simulink model "ARC_DTm"  (R2025b)
settings: Solver=FixedStepAuto  StartTime=0.0  StopTime=10080  FixedStep=1  RelTol=1e-3
PreLoadFcn:
  | %For Preload, set the working path
  | modelFolder = fileparts(which(bdroot));
  | addpath(genpath(modelFolder));
StartFcn:
  | tic
StopFcn:
  | fprintf("Sim Time: %.02f min", toc/60)
values from neighbouring files (symbols this model uses):
  batteryScenario = p.batteryScenario    [RUNSIM_ParameterSweep.m]    (also in _RUNSIM_ParameterSweep.m)
  Electricity_SalePriceModifier = 50/100    (= 0.5)    [RUNSIM_ParameterSweep.m]    (also in _RUNSIM_ParameterSweep.m)
  LUT = LUT_load.gamLUT    [RUNSIM_ParameterSweep.m]    (also in _RUNSIM_ParameterSweep.m)
  minimum_UF_system_flow = 5833    [RUNSIM_ParameterSweep.m]    (also in _RUNSIM_ParameterSweep.m)
  PROS1_recoveryrate = 61    [RUNSIM_ParameterSweep.m]    (also in _RUNSIM_ParameterSweep.m)
  PROS2_recoveryrate = 62    [RUNSIM_ParameterSweep.m]    (also in _RUNSIM_ParameterSweep.m)
  ROstabilization_time = p.ROstabilization_time    [RUNSIM_ParameterSweep.m]    (also in _RUNSIM_ParameterSweep.m)
  solarModifier = maximum_solar_generation / 300    [RUNSIM_ParameterSweep.m]    (also in _RUNSIM_ParameterSweep.m)
  TSRO_recoveryrate = 51    [RUNSIM_ParameterSweep.m]    (also in _RUNSIM_ParameterSweep.m)
  UF_RecoveryRate = 96    [RUNSIM_ParameterSweep.m]    (also in _RUNSIM_ParameterSweep.m)
undefined symbols (not defined in the file or in its folder): A_PROS1, A_PROS2, A_TSRO, B_PROS1, B_PROS2, B_TSRO, BW_Max_Time, BW_Max_Vol_gal, CEB_Max_Time, CEB_Max_Vol_gal, CIP_Max_Time, E, FF, h, L, w
libraries: simulink x40
(part 4 of 11)

== system ARC_DTm/TSRO_2 ==
  note: Units needed:
      | u = cm/sec
      | dh = cm
      | Concentrations = g/L
      | Jw_prev = L/m2/min
      |  = Q (Lpm) / Atot(m2)
      | T = oC
      | q = cm/sec =
      | Q (m3/sec) / Atot (m2)
  Inflow : Inport
  Brine Flow (gpm) : Sum  Inputs=-+
  Bus Creator : BusCreator  Inputs=2
  Bus Creator1 : BusCreator  Inputs=3
  Bus Selector : BusSelector  OutputSignals=TSRO Feed Pressure _Bar,Feed Temperature (oC),TSRO_FeedTDS_gL,TSRO_2_FeedFlow_gpm
  Bus Selector1 : BusSelector  OutputSignals=TSRO_A,TSRO_B,TSRO_Area_m2
  Channel Area (m2) : Product  Inputs=4
  Check Valve : Saturate  UpperLimit=Inf  LowerLimit=0
  Check Valve1 : Saturate  UpperLimit=Inf  LowerLimit=0
  Elements per Vessel : Constant  Value=7
  Feed Channel Height (m) : Constant  Value=L
  Fouling Factor : Constant  Value=1-FF
  Gain : Gain  Gain=3.785
  Initial units : Gain  Gain=10^-8
  Jw_Previous : Memory  InitialCondition=.2949
  "L -> gal" : Gain  Gain=1/3.785
  L>m3 : Gain  Gain=1/1000
  MATLAB Function1 : MATLAB Function  TreatAsAtomicUnit=on
  MATLAB Function2 : MATLAB Function  TreatAsAtomicUnit=on
  Membrane Width (m) : Constant  Value=w
  Min : MinMax  Inputs=2
  Minus : Sum  Inputs=+-|
  Number of Vessels : Constant  Value=15
  Pa > Bar : Gain  Gain=100000
  Permeate Flow (gpm) : Product
  Product : Product  Inputs=*/
  Product2 : Product
  Q (L/min) : Gain  Gain=3.785
  Saturation : Saturate  UpperLimit=Inf  LowerLimit=0
  Scope : Scope
      settings: ActiveDisplayYMinimum=-1  ActiveDisplayYMaximum=1  DataLoggingVariableName=ScopeData76
  Scope1 : Scope
      settings: ActiveDisplayYMinimum=-188.84815571077934  ActiveDisplayYMaximum=426.44465787754609  DataLoggingVariableName=ScopeData31
  Scope2 : Scope
      settings: ActiveDisplayYMinimum=-90.1269420343778  ActiveDisplayYMaximum=348.14455140240847  DataLoggingVariableName=ScopeData32
  Spacer Thickness (mm) : Constant  Value=h
  Subsystem : Subsystem
  bar>psi : Gain  Gain=1/.069
  cperm_previous : Memory  InitialCondition=.008
  gpm > L : Gain  Gain=3.785
  initial Units : Gain  Gain=10^-11
  m/min > cm/sec : Gain  Gain=100/60
  m3 > L : Gain  Gain=1000
  m3 > L1 : Gain  Gain=1000
  m>cm : Gain  Gain=100
  m>mm : Gain  Gain=1000
  mm>  cm : Gain  Gain=.1
  mm>m : Gain  Gain=.001
  psi to Bar : Gain  Gain=.069
  s > min : Gain  Gain=60
  s > min1 : Gain  Gain=60
  TSRO_Permeate : Outport
  TSRO_Brine : Outport  Port=2
  tag scope: TSRO_2_deltaPi=global
  wires:
  m/min > cm/sec/1 -> Subsystem/11(u)
  [TSRO_MembraneConstants] -> Bus Selector1/1
  m3 > L1/1 -> s > min1/1
  Bus Selector/1 -> Min/1, Scope/1, bar>psi/1, Subsystem/2(<S2 Feed Pressure (bar)>)  "<TSRO Feed Pressure _Bar>"
  Bus Selector1/3 -> Permeate Flow (gpm)/2  "<TSRO_Area_m2>"
  Membrane Width (m)/1 -> Channel Area (m2)/1, m>mm/1
  [RO_PermeatePressure] -> psi to Bar/1  "Permeate Pressure (psi)"
  Inflow/1 -> Bus Selector/1
  Bus Selector1/1 -> initial Units/1  "<TSRO_A>"
  Bus Selector1/2 -> Initial units/1  "<TSRO_B>"
  Permeate Flow (gpm)/1 -> Check Valve/1  "TSRO_2_PermeateFlow_gpm"
  Bus Selector/2 -> Subsystem/1(<Feed Temperature (oC)>)  "<Feed Temperature (oC)>"
  Bus Selector/3 -> MATLAB Function2/5(cfeed), Subsystem/6(<S2 Feed Salinity (g/L)>)  "<TSRO_FeedTDS_gL>"
  Bus Selector/4 -> Brine Flow (gpm)/2, Q (L/min)/1  "<TSRO_2_FeedFlow_gpm>"
  Product/1 -> m/min > cm/sec/1
  psi to Bar/1 -> Min/2  "Pressure (bar)"
  MATLAB Function2/1(cbrine) -> Bus Creator1/2  "TSRO_2_BrineConductivity_gL"
  initial Units/1 -> m3 > L/1
  Initial units/1 -> m3 > L1/1
  Spacer Thickness (mm)/1 -> MATLAB Function1/2(h), mm>m/1
  m3 > L/1 -> s > min/1
  Min/1 -> Subsystem/3(Pperm)
  mm>m/1 -> Channel Area (m2)/2
  Channel Area (m2)/1 -> Product/2
  Q (L/min)/1 -> MATLAB Function2/4(Qfeed), L>m3/1  "Qtot (L/min)"
  Bus Creator/1 -> Scope2/1, TSRO_Permeate/1  "PRO1_PermeateFlow"
  Number of Vessels/1 -> Channel Area (m2)/3
  s > min/1 -> Pa > Bar/1
  Elements per Vessel/1 -> Channel Area (m2)/4
  s > min1/1 -> Subsystem/5(Salt Perm (L/m2/min))  "Salt Perm (L/m2/min)"
  Fouling Factor/1 -> Product2/2
  m>mm/1 -> MATLAB Function1/1(W)
  L>m3/1 -> Product/1
  Pa > Bar/1 -> Product2/1  "Water Perm (L/m2/min/Bar)"
  MATLAB Function1/1(dh) -> mm>  cm/1
  Feed Channel Height (m)/1 -> m>cm/1
  Jw_Previous/1 -> Subsystem/8(Jw)  "Jw"
  cperm_previous/1 -> Subsystem/7(cperm)  "cperm"
  m>cm/1 -> Subsystem/10(L)
  Product2/1 -> Subsystem/4(Water Perm (L/m2/min/Bar))  "Water Perm (L/m2/min/Bar)"
  Gain/1 -> MATLAB Function2/2(Qperm)  "Predicted Permeate Flow (L/min)"
  mm>  cm/1 -> Subsystem/9(dh)
  Bus Creator1/1 -> Scope1/1, TSRO_Brine/1  "TSRO_Feedwater"
  bar>psi/1 -> Minus/1  "TSRO_2_ConcentratePressure_psi"
  Subsystem/1(Permeate Flux Rate (L/min/m2)) -> Jw_Previous/1, "L -> gal"/1  "Permeate Flux Rate* (L/min.m2)"
  Subsystem/2(Permeate Salinity g/L) -> Bus Creator/2, MATLAB Function2/1(cperm), cperm_previous/1  "TSRO_2_PermeateSalinity_gL"
  "L -> gal"/1 -> Permeate Flow (gpm)/1
  Subsystem/3(deltaPi_bar) -> [TSRO_2_deltaPi]
  Brine Flow (gpm)/1 -> Check Valve1/1  "TSRO_2_BrineFlow_gpm"
  gpm > L/1 -> MATLAB Function2/3(Qbrine)
  [TSRO_Suction_PressureDrop_psi] -> Minus/2
  Minus/1 -> Bus Creator1/3  "TSRO_2_ConcentratePressure_psi"
  Check Valve1/1 -> Bus Creator1/1, gpm > L/1  "TSRO_2_BrineFlow_gpm"
  Check Valve/1 -> Brine Flow (gpm)/1, Bus Creator/1, Gain/1  "TSRO_2_PermeateFlow_gpm"

== system ARC_DTm/TSRO_3 ==
  note: Units needed:
      | u = cm/sec
      | dh = cm
      | Concentrations = g/L
      | Jw_prev = L/m2/min
      |  = Q (Lpm) / Atot(m2)
      | T = oC
      | q = cm/sec =
      | Q (m3/sec) / Atot (m2)
  Inflow : Inport
  Brine Flow (gpm) : Sum  Inputs=-+
  Bus Creator : BusCreator  Inputs=2
  Bus Creator1 : BusCreator  Inputs=3
  Bus Selector : BusSelector  OutputSignals=TSRO Feed Pressure _Bar,Feed Temperature (oC),TSRO_FeedTDS_gL,TSRO_3_FeedFlow_gpm
  Bus Selector1 : BusSelector  OutputSignals=TSRO_A,TSRO_B,TSRO_Area_m2
  Channel Area (m2) : Product  Inputs=4
  Check Valve : Saturate  UpperLimit=Inf  LowerLimit=0
  Check Valve1 : Saturate  UpperLimit=Inf  LowerLimit=0
  Elements per Vessel : Constant  Value=7
  Feed Channel Height (m) : Constant  Value=L
  Fouling Factor : Constant  Value=1-FF
  Gain : Gain  Gain=3.785
  Initial units : Gain  Gain=10^-8
  Jw_Previous : Memory  InitialCondition=.2949
  "L -> gal" : Gain  Gain=1/3.785
  L>m3 : Gain  Gain=1/1000
  MATLAB Function1 : MATLAB Function  TreatAsAtomicUnit=on
  MATLAB Function2 : MATLAB Function  TreatAsAtomicUnit=on
  Membrane Width (m) : Constant  Value=w
  Min : MinMax  Inputs=2
  Minus : Sum  Inputs=+-|
  Number of Vessels : Constant  Value=15
  Pa > Bar : Gain  Gain=100000
  Permeate Flow (gpm) : Product
  Product : Product  Inputs=*/
  Product2 : Product
  Q (L/min) : Gain  Gain=3.785
  Scope : Scope
      settings: ActiveDisplayYMinimum=-1  ActiveDisplayYMaximum=1  DataLoggingVariableName=ScopeData76
  Scope1 : Scope
      settings: ActiveDisplayYMinimum=-188.84815571077934  ActiveDisplayYMaximum=426.44465787754609  DataLoggingVariableName=ScopeData31
  Scope2 : Scope
      settings: ActiveDisplayYMinimum=-90.1269420343778  ActiveDisplayYMaximum=348.14455140240847  DataLoggingVariableName=ScopeData32
  Spacer Thickness (mm) : Constant  Value=h
  Subsystem : Subsystem
  bar>psi : Gain  Gain=1/.069
  cperm_previous : Memory  InitialCondition=.008
  gpm > L : Gain  Gain=3.785
  initial Units : Gain  Gain=10^-11
  m/min > cm/sec : Gain  Gain=100/60
  m3 > L : Gain  Gain=1000
  m3 > L1 : Gain  Gain=1000
  m>cm : Gain  Gain=100
  m>mm : Gain  Gain=1000
  mm>  cm : Gain  Gain=.1
  mm>m : Gain  Gain=.001
  psi to Bar : Gain  Gain=.069
  s > min : Gain  Gain=60
  s > min1 : Gain  Gain=60
  TSRO_Permeate : Outport
  TSRO_Brine : Outport  Port=2
  tag scope: TSRO_3_deltaPi=global
  wires:
  m/min > cm/sec/1 -> Subsystem/11(u)
  [TSRO_MembraneConstants] -> Bus Selector1/1
  m3 > L1/1 -> s > min1/1
  Bus Selector/1 -> Min/1, Scope/1, bar>psi/1, Subsystem/2(<S2 Feed Pressure (bar)>)  "<TSRO Feed Pressure _Bar>"
  Bus Selector1/3 -> Permeate Flow (gpm)/2  "<TSRO_Area_m2>"
  Membrane Width (m)/1 -> Channel Area (m2)/1, m>mm/1
  [RO_PermeatePressure] -> psi to Bar/1  "Permeate Pressure (psi)"
  Inflow/1 -> Bus Selector/1
  Bus Selector1/1 -> initial Units/1  "<TSRO_A>"
  Bus Selector1/2 -> Initial units/1  "<TSRO_B>"
  Permeate Flow (gpm)/1 -> Check Valve1/1  "TSRO_3_PermeateFlow_gpm"
  Bus Selector/2 -> Subsystem/1(<Feed Temperature (oC)>)  "<Feed Temperature (oC)>"
  Bus Selector/3 -> MATLAB Function2/5(cfeed), Subsystem/6(<S2 Feed Salinity (g/L)>)  "<TSRO_FeedTDS_gL>"
  Bus Selector/4 -> Brine Flow (gpm)/2, Q (L/min)/1  "<TSRO_3_FeedFlow_gpm>"
  Product/1 -> m/min > cm/sec/1
  psi to Bar/1 -> Min/2  "Pressure (bar)"
  MATLAB Function2/1(cbrine) -> Bus Creator1/2  "TSRO_3_BrineConductivity_gL"
  initial Units/1 -> m3 > L/1
  Initial units/1 -> m3 > L1/1
  Spacer Thickness (mm)/1 -> MATLAB Function1/2(h), mm>m/1
  m3 > L/1 -> s > min/1
  Min/1 -> Subsystem/3(Pperm)
  mm>m/1 -> Channel Area (m2)/2
  Channel Area (m2)/1 -> Product/2
  Q (L/min)/1 -> MATLAB Function2/4(Qfeed), L>m3/1  "Qtot (L/min)"
  Bus Creator/1 -> Scope2/1, TSRO_Permeate/1  "PRO1_PermeateFlow"
  Number of Vessels/1 -> Channel Area (m2)/3
  s > min/1 -> Pa > Bar/1
  Elements per Vessel/1 -> Channel Area (m2)/4
  s > min1/1 -> Subsystem/5(Salt Perm (L/m2/min))  "Salt Perm (L/m2/min)"
  Fouling Factor/1 -> Product2/2
  m>mm/1 -> MATLAB Function1/1(W)
  L>m3/1 -> Product/1
  Pa > Bar/1 -> Product2/1  "Water Perm (L/m2/min/Bar)"
  MATLAB Function1/1(dh) -> mm>  cm/1
  Feed Channel Height (m)/1 -> m>cm/1
  Jw_Previous/1 -> Subsystem/8(Jw)  "Jw"
  cperm_previous/1 -> Subsystem/7(cperm)  "cperm"
  m>cm/1 -> Subsystem/10(L)
  Product2/1 -> Subsystem/4(Water Perm (L/m2/min/Bar))  "Water Perm (L/m2/min/Bar)"
  Gain/1 -> MATLAB Function2/2(Qperm)  "Predicted Permeate Flow (L/min)"
  mm>  cm/1 -> Subsystem/9(dh)
  Bus Creator1/1 -> Scope1/1, TSRO_Brine/1  "TSRO_Feedwater"
  bar>psi/1 -> Minus/1  "TSRO_3_ConcentratePressure_psi"
  Subsystem/1(Permeate Flux Rate (L/min/m2)) -> Jw_Previous/1, "L -> gal"/1  "Permeate Flux Rate* (L/min.m2)"
  Subsystem/2(Permeate Salinity g/L) -> Bus Creator/2, MATLAB Function2/1(cperm), cperm_previous/1  "TSRO_3_PermeateSalinity_gL"
  "L -> gal"/1 -> Permeate Flow (gpm)/1
  Subsystem/3(deltaPi_bar) -> [TSRO_3_deltaPi]
  Check Valve/1 -> gpm > L/1, Bus Creator1/1  "TSRO_3_BrineFlow_gpm"
  gpm > L/1 -> MATLAB Function2/3(Qbrine)
  [TSRO_Suction_PressureDrop_psi] -> Minus/2
  Minus/1 -> Bus Creator1/3  "TSRO_3_ConcentratePressure_psi"
  Brine Flow (gpm)/1 -> Check Valve/1  "TSRO_3_BrineFlow_gpm"
  Check Valve1/1 -> Brine Flow (gpm)/1, Bus Creator/1, Gain/1  "TSRO_3_PermeateFlow_gpm"

== system ARC_DTm/TSRO_4 ==
  note: Units needed:
      | u = cm/sec
      | dh = cm
      | Concentrations = g/L
      | Jw_prev = L/m2/min
      |  = Q (Lpm) / Atot(m2)
      | T = oC
      | q = cm/sec =
      | Q (m3/sec) / Atot (m2)
  Inflow : Inport
  Brine Flow (gpm) : Sum  Inputs=-+
  Bus Creator : BusCreator  Inputs=2
  Bus Creator1 : BusCreator  Inputs=3
  Bus Selector : BusSelector  OutputSignals=TSRO Feed Pressure _Bar,Feed Temperature (oC),TSRO_FeedTDS_gL,TSRO_4_FeedFlow_gpm
  Bus Selector1 : BusSelector  OutputSignals=TSRO_A,TSRO_B,TSRO_Area_m2
  Channel Area (m2) : Product  Inputs=4
  Check Valve : Saturate  UpperLimit=Inf  LowerLimit=0
  Check Valve1 : Saturate  UpperLimit=Inf  LowerLimit=0
  Elements per Vessel : Constant  Value=7
  Feed Channel Height (m) : Constant  Value=L
  Fouling Factor : Constant  Value=1-FF
  Gain : Gain  Gain=3.785
  Initial units : Gain  Gain=10^-8
  Jw_Previous : Memory  InitialCondition=.2949
  "L -> gal" : Gain  Gain=1/3.785
  L>m3 : Gain  Gain=1/1000
  MATLAB Function1 : MATLAB Function  TreatAsAtomicUnit=on
  MATLAB Function2 : MATLAB Function  TreatAsAtomicUnit=on
  Membrane Width (m) : Constant  Value=w
  Min : MinMax  Inputs=2
  Minus : Sum  Inputs=+-|
  Number of Vessels : Constant  Value=15
  Pa > Bar : Gain  Gain=100000
  Permeate Flow (gpm) : Product
  Product : Product  Inputs=*/
  Product2 : Product
  Q (L/min) : Gain  Gain=3.785
  Scope : Scope
      settings: ActiveDisplayYMinimum=-1  ActiveDisplayYMaximum=1  DataLoggingVariableName=ScopeData76
  Scope1 : Scope
      settings: ActiveDisplayYMinimum=-106.05017960921796  ActiveDisplayYMaximum=153.48557143336205  DataLoggingVariableName=ScopeData31
  Scope2 : Scope
      settings: ActiveDisplayYMinimum=-90.1269420343778  ActiveDisplayYMaximum=348.14455140240847  DataLoggingVariableName=ScopeData32
  Spacer Thickness (mm) : Constant  Value=h
  Subsystem : Subsystem
  bar>psi : Gain  Gain=1/.069
  cperm_previous : Memory  InitialCondition=.008
  gpm > L : Gain  Gain=3.785
  initial Units : Gain  Gain=10^-11
  m/min > cm/sec : Gain  Gain=100/60
  m3 > L : Gain  Gain=1000
  m3 > L1 : Gain  Gain=1000
  m>cm : Gain  Gain=100
  m>mm : Gain  Gain=1000
  mm>  cm : Gain  Gain=.1
  mm>m : Gain  Gain=.001
  psi to Bar : Gain  Gain=.069
  s > min : Gain  Gain=60
  s > min1 : Gain  Gain=60
  TSRO_Permeate : Outport
  TSRO_Brine : Outport  Port=2
  tag scope: TSRO_4_deltaPi=global
  wires:
  m/min > cm/sec/1 -> Subsystem/11(u)
  [TSRO_MembraneConstants] -> Bus Selector1/1
  m3 > L1/1 -> s > min1/1
  Bus Selector/1 -> Min/1, Scope/1, bar>psi/1, Subsystem/2(<S2 Feed Pressure (bar)>)  "<TSRO Feed Pressure _Bar>"
  Bus Selector1/3 -> Permeate Flow (gpm)/2  "<TSRO_Area_m2>"
  Membrane Width (m)/1 -> Channel Area (m2)/1, m>mm/1
  [RO_PermeatePressure] -> psi to Bar/1  "Permeate Pressure (psi)"
  Inflow/1 -> Bus Selector/1
  Bus Selector1/1 -> initial Units/1  "<TSRO_A>"
  Bus Selector1/2 -> Initial units/1  "<TSRO_B>"
  Permeate Flow (gpm)/1 -> Check Valve1/1  "TSRO_4_PermeateFlow_gpm"
  Bus Selector/2 -> Subsystem/1(<Feed Temperature (oC)>)  "<Feed Temperature (oC)>"
  Bus Selector/3 -> MATLAB Function2/5(cfeed), Subsystem/6(<S2 Feed Salinity (g/L)>)  "<TSRO_FeedTDS_gL>"
  Bus Selector/4 -> Brine Flow (gpm)/2, Q (L/min)/1  "<TSRO_4_FeedFlow_gpm>"
  Product/1 -> m/min > cm/sec/1
  psi to Bar/1 -> Min/2  "Pressure (bar)"
  MATLAB Function2/1(cbrine) -> Bus Creator1/2  "TSRO_4_BrineConductivity_gL"
  initial Units/1 -> m3 > L/1
  Initial units/1 -> m3 > L1/1
  Spacer Thickness (mm)/1 -> MATLAB Function1/2(h), mm>m/1
  m3 > L/1 -> s > min/1
  Min/1 -> Subsystem/3(Pperm)
  mm>m/1 -> Channel Area (m2)/2
  Channel Area (m2)/1 -> Product/2
  Q (L/min)/1 -> MATLAB Function2/4(Qfeed), L>m3/1  "Qtot (L/min)"
  Bus Creator/1 -> Scope2/1, TSRO_Permeate/1  "PRO1_PermeateFlow"
  Number of Vessels/1 -> Channel Area (m2)/3
  s > min/1 -> Pa > Bar/1
  Elements per Vessel/1 -> Channel Area (m2)/4
  s > min1/1 -> Subsystem/5(Salt Perm (L/m2/min))  "Salt Perm (L/m2/min)"
  Fouling Factor/1 -> Product2/2
  m>mm/1 -> MATLAB Function1/1(W)
  L>m3/1 -> Product/1
  Pa > Bar/1 -> Product2/1  "Water Perm (L/m2/min/Bar)"
  MATLAB Function1/1(dh) -> mm>  cm/1
  Feed Channel Height (m)/1 -> m>cm/1
  Jw_Previous/1 -> Subsystem/8(Jw)  "Jw"
  cperm_previous/1 -> Subsystem/7(cperm)  "cperm"
  m>cm/1 -> Subsystem/10(L)
  Product2/1 -> Subsystem/4(Water Perm (L/m2/min/Bar))  "Water Perm (L/m2/min/Bar)"
  Gain/1 -> MATLAB Function2/2(Qperm)  "Predicted Permeate Flow (L/min)"
  mm>  cm/1 -> Subsystem/9(dh)
  Bus Creator1/1 -> Scope1/1, TSRO_Brine/1  "TSRO_Feedwater"
  bar>psi/1 -> Minus/1  "TSRO_4_ConcentratePressure_psi"
  Subsystem/1(Permeate Flux Rate (L/min/m2)) -> Jw_Previous/1, "L -> gal"/1  "Permeate Flux Rate* (L/min.m2)"
  Subsystem/2(Permeate Salinity g/L) -> Bus Creator/2, MATLAB Function2/1(cperm), cperm_previous/1  "TSRO_4_PermeateSalinity_gL"
  "L -> gal"/1 -> Permeate Flow (gpm)/1
  Subsystem/3(deltaPi_bar) -> [TSRO_4_deltaPi]
  Check Valve/1 -> Bus Creator1/1, gpm > L/1  "TSRO_4_BrineFlow_gpm"
  gpm > L/1 -> MATLAB Function2/3(Qbrine)
  [TSRO_Suction_PressureDrop_psi] -> Minus/2
  Minus/1 -> Bus Creator1/3  "TSRO_4_ConcentratePressure_psi"
  Brine Flow (gpm)/1 -> Check Valve/1  "TSRO_4_BrineFlow_gpm"
  Check Valve1/1 -> Brine Flow (gpm)/1, Bus Creator/1, Gain/1  "TSRO_4_PermeateFlow_gpm"

== system ARC_DTm/TSRO_Pump_1 ==
  note: Determine Needed Added Pressure
  note: gpm / (gpm/psi*ft2) / ft2
  S2 Feed Flow Rate (gpm) : Inport
  Bar > psi : Gain  Gain=1/.069
  Bus Creator : BusCreator  Inputs=4
  Bus Selector : BusSelector  OutputSignals=TSRO_A,TSRO_Area_m2
  Bus Selector1 : BusSelector  OutputSignals=TSRO_1_FeedFlow_gpm,TSRO_FeedTDS_gL,TSRO_SuctionPressure_psi
  Constant : Constant  Value=0
  Display : Display
  Display2 : Display
  Gain3 : Gain  Gain=10.76
  MATLAB Function1 : MATLAB Function  TreatAsAtomicUnit=on
  Max : MinMax  Function=max  Inputs=2
  Memory : Memory
  Pa > psi : Gain  Gain=6895
  Product : Product  Inputs=**/
  Product1 : Product
  Scope : Scope  NumInputPorts=3
      settings: ActiveDisplayYMinimum=410.42447825863661  ActiveDisplayYMaximum=523.485280193485  DataLoggingVariableName=ScopeData21
  Scope1 : Scope  NumInputPorts=4
      settings: ActiveDisplayYMinimum=-70.174712486796437  ActiveDisplayYMaximum=115.33681909060641  DataLoggingVariableName=ScopeData24
  Scope2 : Scope
      settings: ActiveDisplayYMinimum=-1  ActiveDisplayYMaximum=1  DataLoggingVariableName=ScopeData18
  Scope3 : Scope
      settings: ActiveDisplayYMinimum=2.9110767702794598  ActiveDisplayYMaximum=3.7356434036475763  DataLoggingVariableName=ScopeData33
  Sum : Sum  Inputs=|-+
  Sum1 : Sum  Inputs=|++
  Sum2 : Sum  Inputs=|++
  m2 > ft2 : Gain  Gain=1/10.76
  m3 > gal : Gain  Gain=264.2
  m3/m2/s/Pa : Gain  Gain=10^-11
  psi to Bar : Gain  Gain=.069
  psi>ft : Gain  Gain=2.31
  s > min : Gain  Gain=60
  TSRO_1_Feedwater : Outport
  tag scope: TSRO_1_Power_kW=global
  wires:
  S2 Feed Flow Rate (gpm)/1 -> Bus Selector1/1  "InflowRate (gpm)"
  Sum1/1 -> Sum2/1  "Net Opposing Pressure (psi)"
  [TSRO_MembraneConstants] -> Bus Selector/1
  Pa > psi/1 -> m2 > ft2/1  "Water Perm (gpm/m2/bar)"
  Sum2/1 -> psi to Bar/1, Sum/2  "TSRO_1_FeedPressure_psi"
  m3 > gal/1 -> s > min/1
  [RO_PermeatePressure] -> Sum1/2
  [T] -> Bus Creator/2  "Feed Temperature (oC)"
  Memory/1 -> Scope1/3, Sum1/1
  Product/1 -> Sum2/2, Scope1/1  "TSRO_1_RequiredNDP_psi"
  psi to Bar/1 -> Bus Creator/4  "TSRO Feed Pressure _Bar"
  Gain3/1 -> Display/1, Product1/2  "TSRO_Area_ft2"
  m2 > ft2/1 -> Product1/1  "TSRO_WaterPermeability_gpm_psi_ft2"
  m3/m2/s/Pa/1 -> m3 > gal/1
  Bus Selector/1 -> m3/m2/s/Pa/1  "<TSRO_A>"
  Product1/1 -> Product/3
  [TSRO_1_deltaPi] -> Scope2/1, Bar > psi/1
  [TSRO_RR] -> Product/2
  s > min/1 -> Pa > psi/1
  Bar > psi/1 -> Memory/1
  Bus Creator/1 -> TSRO_1_Feedwater/1
  psi>ft/1 -> Scope/2, MATLAB Function1/2(h_des)
  Bus Selector1/2 -> Scope3/1, Bus Creator/1  "<TSRO_FeedTDS_gL>"
  Bus Selector1/3 -> Scope1/2, Sum/1  "<TSRO_SuctionPressure_psi>"
  Bus Selector/2 -> Gain3/1  "<TSRO_Area_m2>"
  Bus Selector1/1 -> MATLAB Function1/1(Q_des), Scope/1, Bus Creator/3, Product/1  "<TSRO_1_FeedFlow_gpm>"
  Sum/1 -> Scope1/4, psi>ft/1  "Required added pressure (psi)"
  Max/1 -> [TSRO_1_Power_kW], Display2/1
  Constant/1 -> Max/1
  MATLAB Function1/1(power) -> Max/2, Scope/3  "TSRO_1_Power_kW"

== system ARC_DTm/TSRO_Pump_2 ==
  note: Determine Needed Added Pressure
  note: gpm / (gpm/psi*ft2) / ft2
  S2 Feed Flow Rate (gpm) : Inport
  Bar > psi : Gain  Gain=1/.069
  Bus Creator : BusCreator  Inputs=4
  Bus Selector : BusSelector  OutputSignals=TSRO_A,TSRO_Area_m2
  Bus Selector1 : BusSelector  OutputSignals=TSRO_2_FeedFlow_gpm,TSRO_FeedTDS_gL,TSRO_SuctionPressure_psi
  Constant : Constant  Value=0
  Display : Display
  Display2 : Display
  Gain : Gain  Gain=.01
  Gain3 : Gain  Gain=10.76
  MATLAB Function1 : MATLAB Function  TreatAsAtomicUnit=on
  Max : MinMax  Function=max  Inputs=2
  Memory : Memory
  Pa > psi : Gain  Gain=6895
  Product : Product  Inputs=**/
  Product1 : Product
  Sum : Sum  Inputs=|-+
  Sum1 : Sum  Inputs=|++
  Sum2 : Sum  Inputs=|++
  TSRO_2_recoveryrate_per : Constant  Value=51
  m2 > ft2 : Gain  Gain=1/10.76
  m3 > gal : Gain  Gain=264.2
  m3/m2/s/Pa : Gain  Gain=10^-11
  psi to Bar : Gain  Gain=.069
  psi>ft : Gain  Gain=2.31
  s > min : Gain  Gain=60
  TSRO_2_Feedwater : Outport
  tag scope: TSRO_2_Power_kW=global
  wires:
  S2 Feed Flow Rate (gpm)/1 -> Bus Selector1/1  "InflowRate (gpm)"
  Sum1/1 -> Sum2/1  "Net Opposing Pressure (psi)"
  [TSRO_MembraneConstants] -> Bus Selector/1
  Pa > psi/1 -> m2 > ft2/1  "Water Perm (gpm/m2/bar)"
  Sum2/1 -> psi to Bar/1, Sum/2  "TSRO_2_FeedPressure_psi"
  m3 > gal/1 -> s > min/1
  [RO_PermeatePressure] -> Sum1/2
  [T] -> Bus Creator/2  "Feed Temperature (oC)"
  Memory/1 -> Sum1/1
  Product/1 -> Sum2/2  "TSRO_2_RequiredNDP_psi"
  TSRO_2_recoveryrate_per/1 -> Gain/1
  psi to Bar/1 -> Bus Creator/4  "TSRO Feed Pressure _Bar"
  Gain3/1 -> Display/1, Product1/2  "TSRO_Area_ft2"
  m2 > ft2/1 -> Product1/1  "TSRO_WaterPermeability_gpm_psi_ft2"
  m3/m2/s/Pa/1 -> m3 > gal/1
  Bus Selector/1 -> m3/m2/s/Pa/1  "<TSRO_A>"
  Product1/1 -> Product/3
  [TSRO_2_deltaPi] -> Bar > psi/1
  Gain/1 -> Product/2
  s > min/1 -> Pa > psi/1
  Bar > psi/1 -> Memory/1
  Bus Creator/1 -> TSRO_2_Feedwater/1
  psi>ft/1 -> MATLAB Function1/2(h_des)
  Bus Selector1/2 -> Bus Creator/1  "<TSRO_FeedTDS_gL>"
  Bus Selector1/3 -> Sum/1  "<TSRO_SuctionPressure_psi>"
  Bus Selector/2 -> Gain3/1  "<TSRO_Area_m2>"
  Bus Selector1/1 -> MATLAB Function1/1(Q_des), Bus Creator/3, Product/1  "<TSRO_2_FeedFlow_gpm>"
  Sum/1 -> psi>ft/1
  Max/1 -> Display2/1, [TSRO_2_Power_kW]
  Constant/1 -> Max/1
  MATLAB Function1/1(power) -> Max/2

== system ARC_DTm/TSRO_Pump_3 ==
  note: Determine Needed Added Pressure
  note: gpm / (gpm/psi*ft2) / ft2
  S2 Feed Flow Rate (gpm) : Inport
  Bar > psi : Gain  Gain=1/.069
  Bus Creator : BusCreator  Inputs=4
  Bus Selector : BusSelector  OutputSignals=TSRO_A,TSRO_Area_m2
  Bus Selector1 : BusSelector  OutputSignals=TSRO_3_FeedFlow_gpm,TSRO_FeedTDS_gL,TSRO_SuctionPressure_psi
  Constant : Constant  Value=0
  Display : Display
  Display2 : Display
  Gain : Gain  Gain=.01
  Gain3 : Gain  Gain=10.76
  MATLAB Function1 : MATLAB Function  TreatAsAtomicUnit=on
  Max : MinMax  Function=max  Inputs=2
  Memory : Memory
  Pa > psi : Gain  Gain=6895
  Product : Product  Inputs=**/
  Product1 : Product
  Sum : Sum  Inputs=|-+
  Sum1 : Sum  Inputs=|++
  Sum2 : Sum  Inputs=|++
  TSRO_3_recoveryrate_per : Constant  Value=51
  m2 > ft2 : Gain  Gain=1/10.76
  m3 > gal : Gain  Gain=264.2
  m3/m2/s/Pa : Gain  Gain=10^-11
  psi to Bar : Gain  Gain=.069
  psi>ft : Gain  Gain=2.31
  s > min : Gain  Gain=60
  TSRO_3_Feedwater : Outport
  tag scope: TSRO_3_Power_kW=global
  wires:
  S2 Feed Flow Rate (gpm)/1 -> Bus Selector1/1  "InflowRate (gpm)"
  Sum1/1 -> Sum2/1  "Net Opposing Pressure (psi)"
  [TSRO_MembraneConstants] -> Bus Selector/1
  Pa > psi/1 -> m2 > ft2/1  "Water Perm (gpm/m2/bar)"
  Sum2/1 -> psi to Bar/1, Sum/2  "TSRO_3_FeedPressure_psi"
  m3 > gal/1 -> s > min/1
  [RO_PermeatePressure] -> Sum1/2
  [T] -> Bus Creator/2  "Feed Temperature (oC)"
  Memory/1 -> Sum1/1
  Product/1 -> Sum2/2  "TSRO_3_RequiredNDP_psi"
  TSRO_3_recoveryrate_per/1 -> Gain/1
  psi to Bar/1 -> Bus Creator/4  "TSRO Feed Pressure _Bar"
  Gain3/1 -> Display/1, Product1/2  "TSRO_Area_ft2"
  m2 > ft2/1 -> Product1/1  "TSRO_WaterPermeability_gpm_psi_ft2"
  m3/m2/s/Pa/1 -> m3 > gal/1
  Bus Selector/1 -> m3/m2/s/Pa/1  "<TSRO_A>"
  Product1/1 -> Product/3
  [TSRO_3_deltaPi] -> Bar > psi/1
  Gain/1 -> Product/2
  s > min/1 -> Pa > psi/1
  Bar > psi/1 -> Memory/1
  Bus Creator/1 -> TSRO_3_Feedwater/1
  psi>ft/1 -> MATLAB Function1/2(h_des)
  Bus Selector1/2 -> Bus Creator/1  "<TSRO_FeedTDS_gL>"
  Bus Selector1/3 -> Sum/1  "<TSRO_SuctionPressure_psi>"
  Bus Selector/2 -> Gain3/1  "<TSRO_Area_m2>"
  Bus Selector1/1 -> MATLAB Function1/1(Q_des), Bus Creator/3, Product/1  "<TSRO_3_FeedFlow_gpm>"
  Sum/1 -> psi>ft/1
  Max/1 -> Display2/1, [TSRO_3_Power_kW]
  Constant/1 -> Max/1
  MATLAB Function1/1(power) -> Max/2

== system ARC_DTm/TSRO_Pump_4 ==
  note: Determine Needed Added Pressure
  note: gpm / (gpm/psi*ft2) / ft2
  S2 Feed Flow Rate (gpm) : Inport
  Bar > psi : Gain  Gain=1/.069
  Bus Creator : BusCreator  Inputs=4
  Bus Selector : BusSelector  OutputSignals=TSRO_A,TSRO_Area_m2
  Bus Selector1 : BusSelector  OutputSignals=TSRO_4_FeedFlow_gpm,TSRO_FeedTDS_gL,TSRO_SuctionPressure_psi
  Constant : Constant  Value=0
  Display : Display
  Display2 : Display
  Gain : Gain  Gain=.01
  Gain3 : Gain  Gain=10.76
  MATLAB Function1 : MATLAB Function  TreatAsAtomicUnit=on
  Max : MinMax  Function=max  Inputs=2
  Memory : Memory
  Pa > psi : Gain  Gain=6895
  Product : Product  Inputs=**/
  Product1 : Product
  Sum : Sum  Inputs=|-+
  Sum1 : Sum  Inputs=|++
  Sum2 : Sum  Inputs=|++
  TSRO_4_recoveryrate_per : Constant  Value=51
  m2 > ft2 : Gain  Gain=1/10.76
  m3 > gal : Gain  Gain=264.2
  m3/m2/s/Pa : Gain  Gain=10^-11
  psi to Bar : Gain  Gain=.069
  psi>ft : Gain  Gain=2.31
  s > min : Gain  Gain=60
  TSRO_4_Feedwater : Outport
  tag scope: TSRO_4_Power_kW=global
  wires:
  S2 Feed Flow Rate (gpm)/1 -> Bus Selector1/1  "InflowRate (gpm)"
  Sum1/1 -> Sum2/1  "Net Opposing Pressure (psi)"
  [TSRO_MembraneConstants] -> Bus Selector/1
  Pa > psi/1 -> m2 > ft2/1  "Water Perm (gpm/m2/bar)"
  Sum2/1 -> psi to Bar/1, Sum/2  "TSRO_4_FeedPressure_psi"
  m3 > gal/1 -> s > min/1
  [RO_PermeatePressure] -> Sum1/2
  [T] -> Bus Creator/2  "Feed Temperature (oC)"
  Memory/1 -> Sum1/1
  Product/1 -> Sum2/2  "TSRO_4_RequiredNDP_psi"
  TSRO_4_recoveryrate_per/1 -> Gain/1
  psi to Bar/1 -> Bus Creator/4  "TSRO Feed Pressure _Bar"
  Gain3/1 -> Display/1, Product1/2  "TSRO_Area_ft2"
  m2 > ft2/1 -> Product1/1  "TSRO_WaterPermeability_gpm_psi_ft2"
  m3/m2/s/Pa/1 -> m3 > gal/1
  Bus Selector/1 -> m3/m2/s/Pa/1  "<TSRO_A>"
  Product1/1 -> Product/3
  [TSRO_4_deltaPi] -> Bar > psi/1
  Gain/1 -> Product/2
  s > min/1 -> Pa > psi/1
  Bar > psi/1 -> Memory/1
  Bus Creator/1 -> TSRO_4_Feedwater/1
  psi>ft/1 -> MATLAB Function1/2(h_des)
  Bus Selector1/2 -> Bus Creator/1  "<TSRO_FeedTDS_gL>"
  Bus Selector1/3 -> Sum/1  "<TSRO_SuctionPressure_psi>"
  Bus Selector/2 -> Gain3/1  "<TSRO_Area_m2>"
  Bus Selector1/1 -> MATLAB Function1/1(Q_des), Bus Creator/3, Product/1  "<TSRO_4_FeedFlow_gpm>"
  Sum/1 -> psi>ft/1
  Max/1 -> Display2/1, [TSRO_4_Power_kW]
  Constant/1 -> Max/1
  MATLAB Function1/1(power) -> Max/2

== system ARC_DTm/UF Maintenance Coordinator ==
  Bus Creator{,1..9} (10 alike) : BusCreator  Inputs=2
  Demux : Demux  Outputs=10
  Demux1 : Demux  Outputs=10
  Maint Queue Vector2 : Mux  Inputs=10
  Memory : Memory
  Memory1 : Memory
  Memory2 : Memory
  Sample_Stateflows : Stateflow chart  Commented=on  TreatAsAtomicUnit=on
  Scope1 : Scope  NumInputPorts=3
      settings: ActiveDisplayYMinimum=-1.25  ActiveDisplayYMaximum=1.25
  Scope2 : Scope
      settings: ActiveDisplayYMinimum=-1  ActiveDisplayYMaximum=1  DataLoggingVariableName=ScopeData14
  Scope3 : Scope
      settings: ActiveDisplayYMinimum=-1  ActiveDisplayYMaximum=1  DataLoggingVariableName=ScopeData15
  Scope5 : Scope
      settings: ActiveDisplayYMinimum=-1.2345292012789748  ActiveDisplayYMaximum=1.3904707987210259  DataLoggingVariableName=ScopeData17
  Scope6 : Scope  NumInputPorts=2
      settings: ActiveDisplayYMinimum=-0.12499999999999997  ActiveDisplayYMaximum=1.125  DataLoggingVariableName=ScopeData18
  UF_FIFO_Coordinator : MATLAB Function  Priority=100  TreatAsAtomicUnit=on  SystemSampleTime=1
  UF_State_Tracker : MATLAB Function  TreatAsAtomicUnit=on  SystemSampleTime=1
  arhive : Subsystem
  tag scope: UF10_State=global, UF1_State=global, UF2_State=global, UF3_State=global, UF4_State=global, UF5_State=global, UF6_State=global, UF7_State=global, UF8_State=global, UF9_State=global, UF_Flow_Assignment=global, UF_Operations_States_vector=global
  wires:
  UF_State_Tracker/3(operations_states) -> Scope5/1, [UF_Operations_States_vector], UF_FIFO_Coordinator/3(operating_states)
  UF_State_Tracker/1(in_startup_queue) -> Scope3/1, UF_FIFO_Coordinator/1(startup_req)
  UF_State_Tracker/2(in_maint_queue) -> Scope2/1, UF_FIFO_Coordinator/2(maint_req)
  UF_State_Tracker/4(maintenance_completion_indicators) -> Scope6/1, Scope1/3, [UF_Maintenance_Completion_Signals]  "Maintenance Completion"
  UF_FIFO_Coordinator/1(startup_cmd) -> Memory/1
  UF_FIFO_Coordinator/2(maint_cmd) -> Memory1/1
  Memory/1 -> UF_State_Tracker/1(startup_cmd)
  Memory1/1 -> UF_State_Tracker/2(maint_cmd)
  UF_FIFO_Coordinator/3(shutdown_cmd) -> Memory2/1
  Memory2/1 -> UF_State_Tracker/3(shutdown_cmd)
  [UF2_Maintenance_Request] -> Maint Queue Vector2/2
  [UF3_Maintenance_Request] -> Maint Queue Vector2/3
  [UF7_Maintenance_Request] -> Maint Queue Vector2/7
  [UF8_Maintenance_Request] -> Maint Queue Vector2/8
  [UF5_Maintenance_Request] -> Maint Queue Vector2/5
  [UF6_Maintenance_Request] -> Maint Queue Vector2/6
  [UF10_Maintenance_Request] -> Maint Queue Vector2/10
  [UF9_Maintenance_Request] -> Maint Queue Vector2/9
  [UF4_Maintenance_Request] -> Maint Queue Vector2/4
  [UF1_Maintenance_Request] -> Maint Queue Vector2/1
  [UF_Maintenance_Completion_Signals] -> Demux/1
  Maint Queue Vector2/1 -> Scope6/2, UF_State_Tracker/4(maint_req)
  Demux/1 -> Bus Creator/1  "UF1_MaintenanceCompletion_signal"
  Bus Creator/1 -> [UF1_State]
  Demux/2 -> Bus Creator1/1  "UF2_MaintenanceCompletion_signal"
  Demux/3 -> Bus Creator2/1  "UF3_MaintenanceCompletion_signal"
  Demux/4 -> Bus Creator3/1  "UF4_MaintenanceCompletion_signal"
  Demux/5 -> Bus Creator4/1  "UF5_MaintenanceCompletion_signal"
  Bus Creator1/1 -> [UF2_State]
  Demux/6 -> Bus Creator5/1  "UF6_MaintenanceCompletion_signal"
  Bus Creator3/1 -> [UF4_State]
  Bus Creator2/1 -> [UF3_State]
  Bus Creator5/1 -> [UF6_State]
  Bus Creator4/1 -> [UF5_State]
  Bus Creator7/1 -> [UF8_State]
  Bus Creator6/1 -> [UF7_State]
  Bus Creator9/1 -> [UF10_State]
  Bus Creator8/1 -> [UF9_State]
  Demux/7 -> Bus Creator6/1  "UF7_MaintenanceCompletion_signal"
  Demux/8 -> Bus Creator7/1  "UF8_MaintenanceCompletion_signal"
  Demux/9 -> Bus Creator8/1  "UF9_MaintenanceCompletion_signal"
  Demux/10 -> Bus Creator9/1  "UF10_MaintenanceCompletion_signal"
  Demux1/2 -> Bus Creator1/2  "UF2_OperationsState_signal"
  Demux1/7 -> Bus Creator6/2  "UF7_OperationsState_signal"
  Demux1/10 -> Bus Creator9/2  "UF10_OperationsState_signal"
  Demux1/1 -> Bus Creator/2  "UF1_OperationsState_signal"
  Demux1/8 -> Bus Creator7/2  "UF8_OperationsState_signal"
  Demux1/4 -> Bus Creator3/2  "UF4_OperationsState_signal"
  Demux1/9 -> Bus Creator8/2  "UF9_OperationsState_signal"
  Demux1/3 -> Bus Creator2/2  "UF3_OperationsState_signal"
  [UF_Operations_States_vector] -> Scope1/1, Demux1/1  "OperationsStates"
  Demux1/5 -> Bus Creator4/2  "UF5_OperationsState_signal"
  Demux1/6 -> Bus Creator5/2  "UF6_OperationsState_signal"
  UF_FIFO_Coordinator/4(assigned_flows) -> Scope1/2, [UF_Flow_Assignment]  "Flows"
  [UFMembrane_FlowVector] -> UF_FIFO_Coordinator/4(flows)

== system ARC_DTm/UF Pumping ==
  Autostrainer_HeadLoss_psi : Constant  Value=5
  Bus Creator : BusCreator  Inputs=3
  Bus Selector : BusSelector  OutputSignals=MaxFlow_gpm,MinFlow_gpm
  Bus Selector1 : BusSelector  OutputSignals=Plant Feed Setpoint,Plant Feed Actual
  Display : Display
  Display1 : Display
  MATLAB Function : MATLAB Function  TreatAsAtomicUnit=on
  Memory : Memory
  Memory1 : Memory
  Saturation : Saturate  UpperLimit=11000  LowerLimit=minimum_UF_system_flow
  Saturation1 : Saturate  UpperLimit=11000  LowerLimit=minimum_UF_system_flow
  Scope : Scope  NumInputPorts=4
      settings: ActiveDisplayYMinimum=-11.154361957059978  ActiveDisplayYMaximum=100.38925761353981  DataLoggingVariableName=ScopeData23
  Sum : Sum  Inputs=+-+|
  Sum1 : Sum  Inputs=|-+
  UF_SuctionPressure_psi : Constant  Value=-12
  psi > ft : Gain  Gain=2.31
  UF_Pump_Discharge : Outport
  tag scope: UFPump_FlowperUnit=global, UF_PumpPower_Vector=global
  wires:
  Sum/1 -> Memory1/1  "UF Feed Pressure_psi"
  UF_SuctionPressure_psi/1 -> Sum/2  "S1 Suction Pressure (psi)"
  MATLAB Function/2(powers) -> [UF_PumpPower_Vector], Scope/2  "Predicted Power Consumption (kW)"
  Bus Creator/1 -> UF_Pump_Discharge/1
  [UFPump_FeedPressure_psi] -> Sum/3
  [UF_FeedFlow] -> Scope/4, Bus Selector1/1
  [UFPump_Bounds] -> Bus Selector/1
  Bus Selector/1 -> MATLAB Function/1(max_flow_per_unit)  "<MaxFlow_gpm>"
  MATLAB Function/1(speeds) -> Display/1, Scope/1
  Autostrainer_HeadLoss_psi/1 -> Sum1/1, Sum/1  "Autostrainer Headloss_psi"
  Sum1/1 -> Bus Creator/3  "UF_FeedPressure_psi"
  MATLAB Function/4(flows) -> Scope/3, Memory/1, [UFPump_FlowperUnit], Display1/1  "UF Flow Vector"
  psi > ft/1 -> MATLAB Function/6(h_des)
  Bus Selector1/1 -> Saturation/1  "<Plant Feed Setpoint>"
  Bus Selector1/2 -> Saturation1/1  "<Plant Feed Actual>"
  Memory/1 -> MATLAB Function/5(prev_flows)
  Bus Selector/2 -> MATLAB Function/2(min_flow_per_unit)  "<MinFlow_gpm>"
  Saturation/1 -> Bus Creator/1, MATLAB Function/3(flow_setpoint)  "UFFeedFlow_Setpoint_gpm"
  Saturation1/1 -> Bus Creator/2, MATLAB Function/4(flow_actual)  "UFFeedFlow_Actual_gpm"
  Memory1/1 -> Sum1/2, psi > ft/1

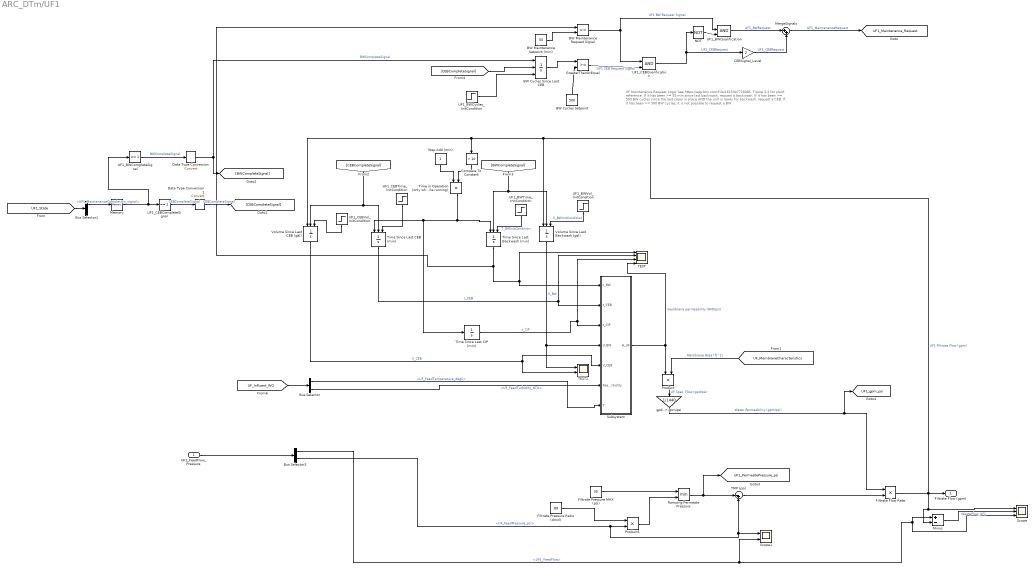
== system ARC_DTm/UF1 ==
  note: UF Maintenance Request Logic
      | See https://app.box.com/file/1615307718366, Figure 3-2 for plant reference.
      |
      | If it has been >= 55 min since last backwash, request a backwash.
      | If it has been >= 500 BW cycles since the last clean in place AND the unit is ready for backwash, request a CEB.
      | If it has been >= 500 BW cycles, it is not possible to request a BW
  UF1_FeedFlow_Pressure : Inport
  BW Cycles Setpoint : Constant  Value=500
  BW Cycles Since Last CEB : Integrator  ExternalReset=rising  InitialConditionSource=external  InitialCondition=5
  BW Maintenance Request Signal : RelationalOperator  OutDataTypeStr=boolean  RndMeth=Simplest  InputSameDT=off
  BW Maintenance Setpoint (min) : Constant  Value=55
  Bus Selector : BusSelector  OutputSignals=UF_FeedTemperature_degC,UF_FeedTurbidity_NTU
  Bus Selector1 : BusSelector  OutputSignals=UF1_MaintenanceCompletion_signal,UF1_OperationsState_signal
  Bus Selector3 : BusSelector  OutputSignals=UF1_FeedFlow,UF_FeedPressure_psi
  CEBSignal_Level : Gain  Gain=2  OutDataTypeStr=double
  Compare To Constant : simulink/Logic and Bit Operations/Compare To Constant  relop=>  const=10  OutDataTypeStr=boolean
  Data Type Conversion : DataTypeConversion  SaturateOnIntegerOverflow=off  RndMeth=Floor
  Data Type Conversion1 : DataTypeConversion  SaturateOnIntegerOverflow=off  RndMeth=Floor
  Filtrate Flow Rate : Product
  Filtrate Pressure MAX (psi) : Constant  Value=39
  Filtrate Pressure Ratio (dmnl) : Constant  Value=.89
  GreaterThanOrEqual : RelationalOperator  OutDataTypeStr=boolean  RndMeth=Simplest  InputSameDT=off
  Memory : Memory
  MergeSignals : Sum  Inputs=|++
  Minus : Sum  Inputs=+-
  NOT : Logic  Operator=NOT  IconShape=distinctive  AllPortsSameDT=off  OutDataTypeStr=boolean
  Product : Product
  Product1 : Product
  Ramping Permeate Pressure : MinMax  Inputs=2
  Scope : Scope  NumInputPorts=3
      settings: ActiveDisplayYMinimum=-126.71796384165732  ActiveDisplayYMaximum=1140.4616745749161  DataLoggingVariableName=ScopeData10
  Scope1 : Scope  NumInputPorts=2
      settings: ActiveDisplayYMinimum=-150.54718641955003  ActiveDisplayYMaximum=1637.0052429355055  DataLoggingVariableName=ScopeData11
  Step Add (min) : Constant
  Subsystem : Subsystem
  TEST : Scope  NumInputPorts=4
      settings: ActiveDisplayYMinimum=-612.74999999999989  ActiveDisplayYMaximum=5514.75  DataLoggingVariableName=ScopeData3
  TEST2 : Scope  NumInputPorts=2
      settings: ActiveDisplayYMinimum=-311929.86683332996  ActiveDisplayYMaximum=2.8073688014999703E+6  DataLoggingVariableName=ScopeData4
  TMP (psi) : Sum  Inputs=|-+
  Time Since Last Backwash (min) : Integrator  ExternalReset=level hold  InitialConditionSource=external  InitialCondition=26
  Time Since Last CEB (min) : Integrator  ExternalReset=level hold  InitialConditionSource=external  InitialCondition=4833
  Time Since Last CIP (min) : Integrator  InitialCondition=round(CIP_Max_Time*rand())
  Time in Operation (only while running) : Product
  UF1_BWCompleteSignal : simulink/Logic and Bit Operations/Compare To Constant  relop===  const=1  OutDataTypeStr=uint8
  UF1_BWCycles_InitCondition : Step  Before=round(500 * rand())  After=0  SampleTime=0
  UF1_BWQualification : Logic  IconShape=distinctive  AllPortsSameDT=off  OutDataTypeStr=boolean
  UF1_BWTime_InitCondition : Step  Before=round(BW_Max_Time*rand())  After=0  SampleTime=0
  UF1_BWVol_InitCondition : Step  Before=round(BW_Max_Vol_gal*rand())  After=0  SampleTime=0
  UF1_CEBCompleteSignal : simulink/Logic and Bit Operations/Compare To Constant  relop===  const=2  OutDataTypeStr=uint8
  UF1_CEBQualification : Logic  IconShape=distinctive  AllPortsSameDT=off  OutDataTypeStr=boolean
  UF1_CEBTime_InitCondition : Step  Before=round(CEB_Max_Time*rand())  After=0  SampleTime=0
  UF1_CEBVol_InitCondition : Step  Before=round(CEB_Max_Vol_gal*rand())  After=0  SampleTime=0
  Volume Since Last Backwash (gal) : Integrator  ExternalReset=level hold  InitialConditionSource=external  InitialCondition=34330
  Volume Since Last CEB (gal) : Integrator  ExternalReset=rising  InitialConditionSource=external  InitialCondition=2777254
  "gpd -> gpm/psi" : Gain  Gain=1/1440
  Filtrate Flow (gpm) : Outport
  tag scope: UF1_Maintenance_Request=global, UF1_PermeatePressure_psi=global, UF1_gpm_psi=global
  wires:
  Volume Since Last Backwash (gal)/1 -> Subsystem/4(V_BW), TEST2/1  "V_BW"
  Time Since Last Backwash (min)/1 -> BW Maintenance Request Signal/1, Subsystem/1(t_BW), TEST/1
  Product/1 -> "gpd -> gpm/psi"/1  "UF Spec. Flow (gpd/psi)"
  [UF_MembraneCharacteristics] -> Product/2  "Membrane Area (ft^2)"
  "gpd -> gpm/psi"/1 -> Filtrate Flow Rate/1, [UF1_gpm_psi]  "Water Permeability (gpm/psi)"
  Time in Operation (only while running)/1 -> Time Since Last Backwash (min)/1, Time Since Last CEB (min)/1, Time Since Last CIP (min)/1
  Filtrate Flow Rate/1 -> Scope/1, Minus/2, Volume Since Last Backwash (gal)/1, Volume Since Last CEB (gal)/1, Compare To Constant/1, Filtrate Flow (gpm)/1  "UF1 Filtrate Flow (gpm)"
  Time Since Last CEB (min)/1 -> Subsystem/2(t_CEB), TEST/2  "t_CEB"
  Volume Since Last CEB (gal)/1 -> Subsystem/5(V_CEB), TEST2/2  "V_CEB"
  Time Since Last CIP (min)/1 -> Subsystem/3(t_CIP), TEST/3  "t_CIP"
  Filtrate Pressure MAX (psi)/1 -> Ramping Permeate Pressure/1
  [UF_Influent_WQ] -> Bus Selector/1
  Bus Selector/1 -> Subsystem/7(T)  "<UF_FeedTemperature_degC>"
  UF1_FeedFlow_Pressure/1 -> Bus Selector3/1
  Filtrate Pressure Ratio (dmnl)/1 -> Product1/1
  Product1/1 -> Ramping Permeate Pressure/2
  Ramping Permeate Pressure/1 -> [UF1_PermeatePressure_psi], TMP (psi)/1
  TMP (psi)/1 -> Filtrate Flow Rate/2
  BW Maintenance Setpoint (min)/1 -> BW Maintenance Request Signal/2
  BW Cycles Since Last CEB/1 -> GreaterThanOrEqual/1
  BW Cycles Setpoint/1 -> GreaterThanOrEqual/2
  Bus Selector/2 -> Subsystem/6(Feed Turbidity)  "<UF_FeedTurbidity_NTU>"
  [UF1_State] -> Bus Selector1/1
  MergeSignals/1 -> [UF1_Maintenance_Request]  "UF1_MaintenanceRequest"
  UF1_CEBCompleteSignal/1 -> Data Type Conversion1/1  "CEBCompleteSignal"
  [CEBCompleteSignal] -> Volume Since Last CEB (gal)/2, Time Since Last CEB (min)/2
  Data Type Conversion/1 -> [BWCompleteSignal], BW Cycles Since Last CEB/1  "BWCompleteSignal"
  [BWCompleteSignal] -> Volume Since Last Backwash (gal)/2, Time Since Last Backwash (min)/2
  [CEBCompleteSignal] -> BW Cycles Since Last CEB/2
  Bus Selector1/1 -> Memory/1  "<UF1_MaintenanceCompletion_signal>"
  UF1_BWCompleteSignal/1 -> Data Type Conversion/1  "BWCompleteSignal"
  Data Type Conversion1/1 -> [CEBCompleteSignal]  "CEBCompleteSignal"
  UF1_BWCycles_InitCondition/1 -> BW Cycles Since Last CEB/3
  Subsystem/1(A_UF) -> TEST/4, Product/1  "membrane permeability (GFD/psi)"
  UF1_BWTime_InitCondition/1 -> Time Since Last Backwash (min)/3  "T_BWInitCondition"
  UF1_CEBVol_InitCondition/1 -> Volume Since Last CEB (gal)/3
  UF1_CEBTime_InitCondition/1 -> Time Since Last CEB (min)/3
  UF1_BWVol_InitCondition/1 -> Volume Since Last Backwash (gal)/3  "V_BWInitCondition"
  Step Add (min)/1 -> Time in Operation (only while running)/1
  Compare To Constant/1 -> Time in Operation (only while running)/2
  Memory/1 -> UF1_BWCompleteSignal/1, UF1_CEBCompleteSignal/1
  UF1_BWQualification/1 -> MergeSignals/1  "UF1_BWRequest"
  GreaterThanOrEqual/1 -> UF1_CEBQualification/2  "UF1 CEB Request Signal"
  UF1_CEBQualification/1 -> CEBSignal_Level/1, NOT/1  "UF1_CEBRequest"
  BW Maintenance Request Signal/1 -> UF1_BWQualification/1, UF1_CEBQualification/1  "UF1 BW Request Signal"
  NOT/1 -> UF1_BWQualification/2
  CEBSignal_Level/1 -> MergeSignals/2  "UF1_CEBRequest"
  Bus Selector3/1 -> Scope1/2, Minus/1, Scope/3  "<UF1_FeedFlow>"
  Bus Selector3/2 -> TMP (psi)/2, Scope1/1, Product1/2  "<UF_FeedPressure_psi>"
  Minus/1 -> Scope/2  "WasteFlow_UF1"
